simulink model "Fuzzy Controller Simulink Model"  (R2020a)
settings: Solver=VariableStepAuto  StartTime=0.0  StopTime=300  RelTol=1e-3
libraries: fuzblock x1
settings Model: Creator=USER  LastModifiedBy=USER

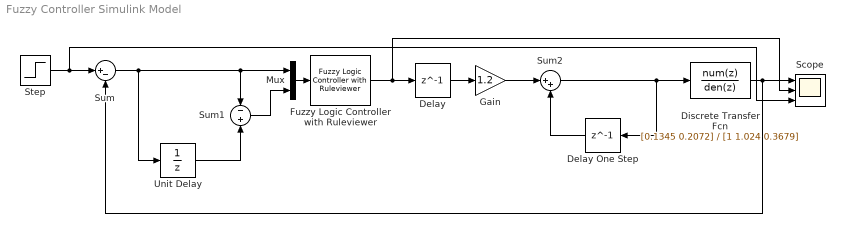
== system Fuzzy Controller Simulink Model ==
  Delay : Delay  DelayLength=1
  Delay One Step : Delay  DelayLength=1
  Discrete Transfer Fcn : DiscreteTransferFcn  Numerator=[0.1345 0.2072]  Denominator=[1 1.024 0.3679]
  Fuzzy Logic Controller with Ruleviewer : fuzblock/Fuzzy Logic  Controller  with Ruleviewer  fismatrix=ETS_SPC  Ts=1
  Gain : Gain  Gain=1.2
  Mux : Mux  Inputs=2
  Scope : Scope  NumInputPorts=3
  Step : Step  After=6  SampleTime=0
  Sum : Sum  Inputs=|+-
  Sum1 : Sum  Inputs=-+
  Sum2 : Sum  Inputs=|++
  Unit Delay : UnitDelay  SampleTime=-1  HasFrameUpgradeWarning=on
  wires:
  Mux/1 -> Fuzzy Logic Controller with Ruleviewer/1
  Sum/1 -> Mux/1, Sum1/1, Unit Delay/1
  Unit Delay/1 -> Sum1/2
  Sum1/1 -> Mux/2
  Discrete Transfer Fcn/1 -> Scope/1, Sum/2
  Fuzzy Logic Controller with Ruleviewer/1 -> Scope/2, Delay/1
  Sum2/1 -> Delay One Step/1, Discrete Transfer Fcn/1
  Delay/1 -> Gain/1
  Gain/1 -> Sum2/1
  Delay One Step/1 -> Sum2/2
  Step/1 -> Scope/3, Sum/1
